simulink model "trim_Lagrangian_Model_Nonlinear_R2009a"  (Simulink 7.3)
settings: Solver=ode45  StartTime=0.0  StopTime=10.0  RelTol=1e-3
libraries: lib_Lagrangian_Model_Nonlinear x1
settings Model: Creator=ottoe  LastModifiedBy=ottoe  CovModelRefEnable=off
settings DataIOCC: LimitDataPoints=off  SaveFormat=StructureWithTime  ReturnWorkspaceOutputs=off
settings OptimizationCC: ExpressionDepthLimit=128
settings DebuggingCC: UnderspecifiedInitializationDetection=Simplified  MergeDetectMultiDrivingBlocksExec=error  SolverPrmCheckMsg=none  FcnCallInpInsideContextMsg=Enable All  StateNameClashWarn=none  StrictBusMsg=ErrorLevel1
settings HardwareCC: ProdIntDivRoundTo=Zero  ProdEndianess=LittleEndian  ProdHWDeviceType=Specified
settings CodeAppCC: CustomSymbolStrType=$N$R$M_T
settings GRTTargetCC: TargetFunctionLibrary=C89/C90 (ANSI)

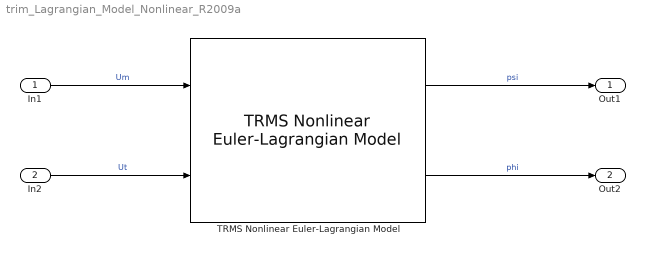
== system trim_Lagrangian_Model_Nonlinear_R2009a ==
  In1 : Inport
  In2 : Inport  Port=2
  TRMS Nonlinear Euler-Lagrangian Model : lib_Lagrangian_Model_Nonlinear/TRMS Nonlinear Euler-Lagrangian Model  Psi_zero=0  Psi_dot_zero=0  Phi_zero=0  Phi_dot_zero=0  Wm_zero=0  Wt_zero=0
  Out1 : Outport
  Out2 : Outport  Port=2
  wires:
  In1/1 -> TRMS Nonlinear Euler-Lagrangian Model/1  "Um"
  In2/1 -> TRMS Nonlinear Euler-Lagrangian Model/2  "Ut"
  TRMS Nonlinear Euler-Lagrangian Model/1 -> Out1/1  "psi"
  TRMS Nonlinear Euler-Lagrangian Model/2 -> Out2/1  "phi"
